simulink model "exp_6"  (R2013b)
settings: Solver=ode45  StartTime=0.0  StopTime=10.0  RelTol=1e-3
libraries: simulink x1
settings Model: Creator=lenovo  LastModifiedBy=lenovo

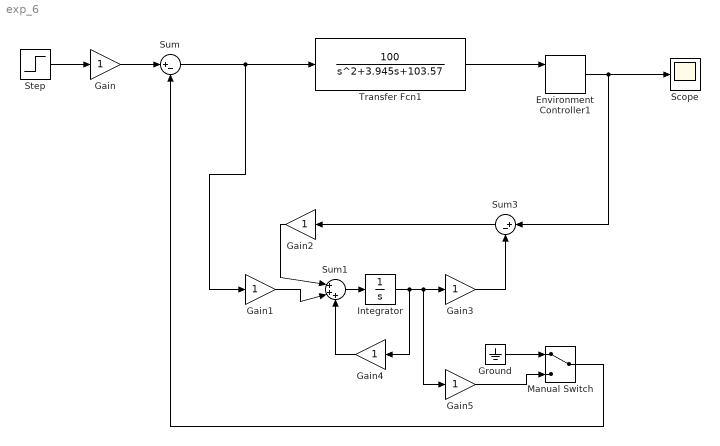
== system exp_6 ==
  Environment Controller1 : simulink/Signal Routing/Environment Controller
  Gain{,1..5} (6 alike) : Gain
  Ground : Ground
  Integrator : Integrator
  Manual Switch : ManualSwitch
  Scope : Scope
  Step : Step  SampleTime=0
  Sum : Sum  Inputs=|+-
  Sum1 : Sum  Inputs=|+++
  Sum3 : Sum  Inputs=|+-
  Transfer Fcn1 : TransferFcn  Numerator=[100]  Denominator=[1 3.945 103.57]
  wires:
  Step/1 -> Gain/1
  Gain/1 -> Sum/1
  Sum/1 -> Gain1/1, Transfer Fcn1/1
  Transfer Fcn1/1 -> Environment Controller1/1
  Environment Controller1/1 -> Sum3/1, Scope/1
  Sum3/1 -> Gain2/1
  Gain2/1 -> Sum1/1
  Gain1/1 -> Sum1/2
  Sum1/1 -> Integrator/1
  Integrator/1 -> Gain4/1, Gain5/1, Gain3/1
  Gain3/1 -> Sum3/2
  Gain4/1 -> Sum1/3
  Ground/1 -> Manual Switch/1
  Gain5/1 -> Manual Switch/2
  Manual Switch/1 -> Sum/2
